simulink subsystem "Baroreflex_HR"  (R2023b)
settings: Solver=VariableStepAuto  StartTime=0.0  StopTime=10.0  RelTol=1e-3
values from neighbouring files (symbols this model uses):
  a = 0.01    [Project2024_params_Group3.m]
  HR_eq = 70    [Project2024_params_Group3.m]    (also in compute_indices.m = mean(HR_data(pre_infusion_indices)))
  tau_1 = 0.01    [Project2024_params_Group3.m]
settings Model: Creator=jamesyeh  LastModifiedBy=jamesyeh

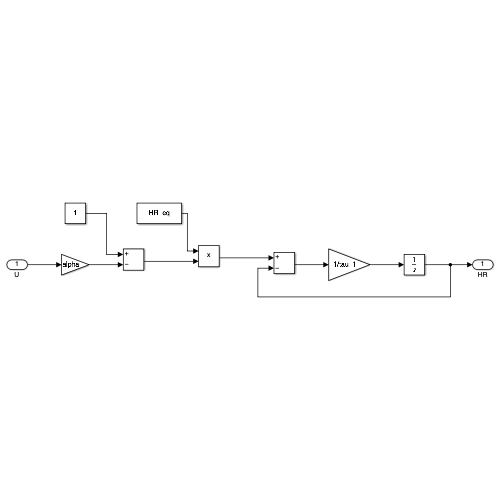
[thumbnail: Simulink's stored preview of the top-level diagram]
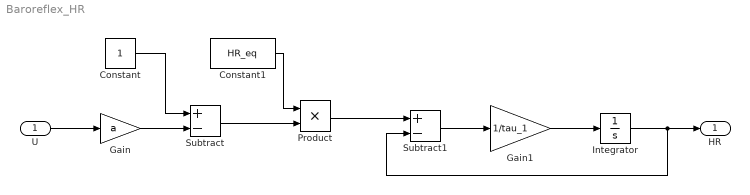
== system Baroreflex_HR ==
  U : Inport
  Constant : Constant
  Constant1 : Constant  Value=HR_eq
  Gain : Gain  Gain=a
  Gain1 : Gain  Gain=1/tau_1
  Integrator : Integrator
  Product : Product
  Subtract : Sum  Inputs=+-
  Subtract1 : Sum  Inputs=+-
  HR : Outport
  wires:
  Constant/1 -> Subtract/1
  Gain/1 -> Subtract/2
  U/1 -> Gain/1
  Constant1/1 -> Product/1
  Subtract/1 -> Product/2
  Product/1 -> Subtract1/1
  Subtract1/1 -> Gain1/1
  Gain1/1 -> Integrator/1
  Integrator/1 -> Subtract1/2, HR/1
